simulink model "uav_control_SMC2"  (R2023a)
settings: Solver=FixedStepAuto  StartTime=0.0  StopTime=100  FixedStep=1e-3
undefined symbols (not defined in the file): c_1, c_2, c_3, c_4, c_5, c_6, c_7, c_8, c_psi, c_z, eps1, eps2, eps3, eps4, eta1, eta2, eta3, eta4, Matrix_Force2angular_velocity
libraries: simulink x18, control_form_LagrangeSimplified x1, control_form_LagrangeSimplified_forces x1
settings Model: Creator=Alex  LastModifiedBy=Alex

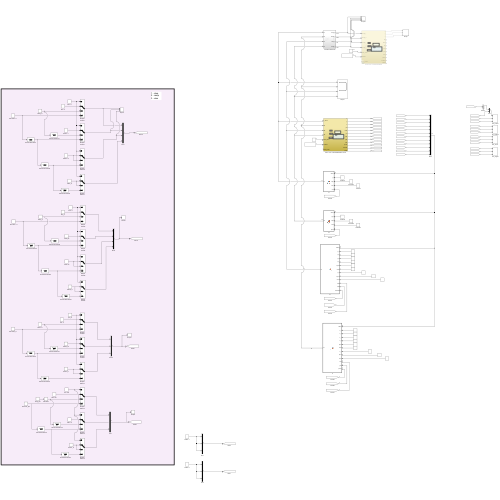
[thumbnail: Simulink's stored preview of the top-level diagram]
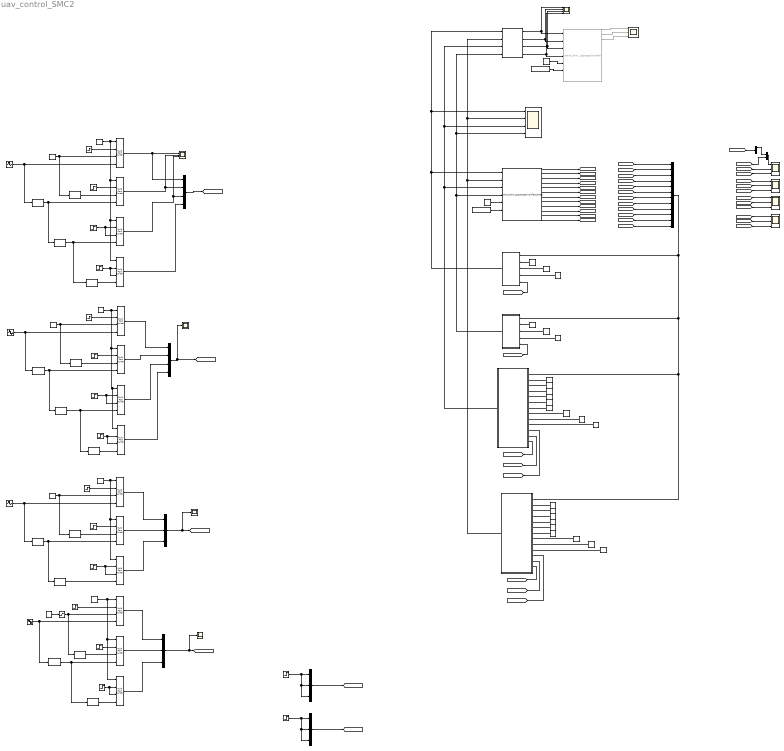
== system uav_control_SMC2 ==
  note: 1 - step
      | 2 - ramp
      | 3 - else
  CNL_AngPos : Scope  NumInputPorts=3
  CNL_AngVel : Scope  NumInputPorts=3
  CNL_LinPos : Scope  NumInputPorts=3
  CNL_LinVel : Scope  NumInputPorts=3
  Constant : Constant  Value=eta1
  Constant1 : Constant  Value=c_z
  Constant10 : Constant  Value=eps3
  Constant11 : Constant  Value=eta3
  Constant12 : Constant  Value=eps4
  Constant13 : Constant  Value=eta4
  Constant14 : Constant  Value=c_5
  Constant15 : Constant  Value=c_6
  Constant16 : Constant  Value=c_7
  Constant17 : Constant  Value=c_8
  Constant18 : Constant  Value=[1 0 0 0 1 1 0]
  Constant19 : Constant  Value=[1 1 -1 0 0 0 0 0 0 0 0 0 ]
  Constant2 : Constant  Value=eps1
  Constant20 : Constant  Value=eta1
  Constant21 : Constant  Value=c_z
  Constant22 : Constant  Value=eps1
  Constant23 : Constant  Value=eta1
  Constant24 : Constant  Value=c_z
  Constant25 : Constant  Value=eps1
  Constant26 : Constant  Value=[1 1 0 0 1 1 0]
  Constant27 : Constant  Value=[1 1 -1 0 0 0 0 0 0 0 0 0 ]
  Constant3 : Constant  Value=eta2
  Constant4 : Constant  Value=c_psi
  Constant5 : Constant  Value=eps2
  Constant6 : Constant  Value=c_1
  Constant7 : Constant  Value=c_2
  Constant8 : Constant  Value=c_3
  Constant9 : Constant  Value=c_4
  Demux : Demux
  Discrete Derivative{3..4,8..9,13..14,18..25} (14 alike) : simulink/Discrete/Discrete Derivative  gainval=1.0  ICPrevScaledInput=0.0  OutMin=[]  OutMax=[]  OutDataType=fixdt(1, 16)  OutScaling=2^-10  DoSatur=off
  Force2AngularVelocity : Subsystem
  Input_psi1 : Constant
  Input_x1 : Constant  Value=2
  Input_y1 : Constant  Value=2
  Input_z1 : Constant  Value=2
  Multiport Switch{3..4,8..9,13..14,18..25} (14 alike) : MultiPortSwitch  SaturateOnIntegerOverflow=off  InputSameDT=off
  Mux : Mux  Inputs=2
  Mux{1,3,9..10} (4 alike) : Mux  Inputs=3
  Mux2 : Mux  Inputs=12
  Mux7 : Mux
  Mux8 : Mux
  Ramp_psi1 : simulink/Sources/Ramp  slope=0.2  start=0  InitialOutput=0
  Ramp_x1 : simulink/Sources/Ramp  slope=1  start=0  InitialOutput=1
  Ramp_y1 : simulink/Sources/Ramp  slope=1  start=0  InitialOutput=0
  Ramp_z1 : simulink/Sources/Ramp  slope=-5  start=0  InitialOutput=0
  STEP0_{1..2,7..8,11..12,15..20} (12 alike) : Step  Time=0  After=0  SampleTime=0
  Saturation1 : Saturate  UpperLimit=pi  LowerLimit=-pi
  Scope : Scope  NumInputPorts=3
  Scope1 : Scope  NumInputPorts=4
  Scope2 : Scope  NumInputPorts=4
  Scope5 : Scope  NumInputPorts=3
  Scope6 : Scope
  Scope7 : Scope
  Scope8 : Scope
  Sine Wave_psi1 : Sin  SampleTime=0
  Sine Wave_x1 : Sin  Frequency=0.5  SampleTime=0
  Sine Wave_y1 : Sin  Amplitude=3  Bias=5  SampleTime=0
  Sine Wave_z1 : Sin  Amplitude=3  Bias=-5  SampleTime=0
  Step_psi1 : Step  Time=0  SampleTime=0
  Step_x1 : Step  Time=0  After=5  SampleTime=0
  Step_y1 : Step  Time=0  After=5  SampleTime=0
  Step_z1 : Step  Time=0  After=-7  SampleTime=0
  control_form_LagrangeSimplified : control_form_LagrangeSimplified/control_form_LagrangeSimplified  Commented=on  SystemSampleTime=-1  VariantActivationTime=update diagram  Latency=0  AutoFrameSizeCalculation=off
  control_form_LagrangeSimplified_forces : control_form_LagrangeSimplified_forces/control_form_LagrangeSimplified_forces  SystemSampleTime=-1  VariantActivationTime=update diagram  Latency=0  AutoFrameSizeCalculation=off
  u1 : MATLAB Function  TreatAsAtomicUnit=on
  u2 : MATLAB Function  TreatAsAtomicUnit=on
  u3 : MATLAB Function  TreatAsAtomicUnit=on
  u4 : MATLAB Function  TreatAsAtomicUnit=on
  wires:
  control_form_LagrangeSimplified_forces/1 -> [CLS_x]
  control_form_LagrangeSimplified_forces/2 -> [CLS_y]
  control_form_LagrangeSimplified_forces/3 -> [CLS_z]
  control_form_LagrangeSimplified_forces/4 -> [CLS_phi]
  control_form_LagrangeSimplified_forces/5 -> [CLS_theta]
  control_form_LagrangeSimplified_forces/6 -> [CLS_psi]
  control_form_LagrangeSimplified_forces/7 -> [CLS_xdot]
  control_form_LagrangeSimplified_forces/8 -> [CLS_ydot]
  control_form_LagrangeSimplified_forces/9 -> [CLS_zdot]
  control_form_LagrangeSimplified_forces/10 -> [CLS_phidot]
  control_form_LagrangeSimplified_forces/11 -> [CLS_thetadot]
  control_form_LagrangeSimplified_forces/12 -> [CLS_psidot]
  [CLS_x] -> Mux/2
  [CLS_y] -> CNL_LinPos/2
  [CLS_z] -> CNL_LinPos/3
  [CLS_theta] -> CNL_AngPos/2
  [CLS_phi] -> CNL_AngPos/1
  [CLS_psi] -> CNL_AngPos/3
  [CLS_xdot] -> CNL_LinVel/1
  [CLS_ydot] -> CNL_LinVel/2
  [CLS_zdot] -> CNL_LinVel/3
  [CLS_psidot] -> CNL_AngVel/3
  [CLS_thetadot] -> CNL_AngVel/2
  [CLS_phidot] -> CNL_AngVel/1
  [CLS_z] -> Mux2/3
  [CLS_psi] -> Mux2/6
  [CLS_zdot] -> Mux2/9
  [CLS_y] -> Mux2/2
  [CLS_theta] -> Mux2/5
  [CLS_ydot] -> Mux2/8
  [CLS_x] -> Mux2/1
  [CLS_phi] -> Mux2/4
  [CLS_xdot] -> Mux2/7
  [CLS_psidot] -> Mux2/12
  [CLS_thetadot] -> Mux2/11
  [CLS_phidot] -> Mux2/10
  [zref] -> u1/5(zref)
  Constant/1 -> u1/4(eta1)
  Constant1/1 -> u1/2(c_z)
  Constant2/1 -> u1/3(eps1)
  Constant5/1 -> u4/3(eps2)
  Constant4/1 -> u4/2(c_psi)
  Constant3/1 -> u4/4(eta2)
  [psiref] -> u4/5(psiref)
  Mux2/1 -> u2/1(states), u3/1(states), u4/1(states), u1/1(states)
  [xref] -> u3/12(xref)
  [thetaref] -> u3/13(thetaref)
  Constant6/1 -> u3/2(c_1)
  Constant7/1 -> u3/3(c_2)
  Constant8/1 -> u3/4(c_3)
  Constant9/1 -> u3/5(c_4)
  Constant10/1 -> u3/6(eps3)
  Constant11/1 -> u3/7(eta3)
  Constant13/1 -> u2/7(eta4)
  Constant12/1 -> u2/6(eps4)
  Constant17/1 -> u2/5(c_8)
  Constant16/1 -> u2/4(c_7)
  Constant15/1 -> u2/3(c_6)
  Constant14/1 -> u2/2(c_5)
  [phiref] -> u2/13(phiref)
  [yref] -> u2/12(yref)
  Constant18/1 -> control_form_LagrangeSimplified_forces/6
  Constant19/1 -> control_form_LagrangeSimplified_forces/5
  Multiport Switch23/1 -> Mux8/1
  Discrete Derivative9/1 -> Multiport Switch9/4, Discrete Derivative13/1
  Sine Wave_psi1/1 -> Discrete Derivative18/1, Multiport Switch14/4
  STEP0_12/1 -> Multiport Switch19/3, Multiport Switch19/2
  Multiport Switch19/1 -> Mux9/3
  Input_psi1/1 -> Multiport Switch19/1, Multiport Switch18/1, Multiport Switch14/1
  STEP0_11/1 -> Multiport Switch18/2
  Saturation1/1 -> Discrete Derivative14/1, Multiport Switch14/3
  Mux10/1 -> Scope7/1, [zref]
  Ramp_psi1/1 -> Saturation1/1
  Discrete Derivative14/1 -> Multiport Switch18/3
  Discrete Derivative23/1 -> Multiport Switch24/3
  Step_y1/1 -> Multiport Switch23/2
  Discrete Derivative18/1 -> Discrete Derivative19/1, Multiport Switch18/4
  Mux9/1 -> Scope8/1, [psiref]
  Discrete Derivative20/1 -> Discrete Derivative21/1, Multiport Switch20/4
  Step_z1/1 -> Multiport Switch8/2
  Discrete Derivative24/1 -> Discrete Derivative25/1, Multiport Switch24/4
  Multiport Switch24/1 -> Mux8/2
  Multiport Switch3/1 -> Mux7/1, Scope5/1
  Step_x1/1 -> Multiport Switch3/2
  STEP0_7/1 -> Multiport Switch4/2
  Multiport Switch4/1 -> Mux7/2, Scope5/2
  Discrete Derivative4/1 -> Multiport Switch4/4, Discrete Derivative20/1
  Discrete Derivative3/1 -> Multiport Switch4/3
  Input_x1/1 -> Multiport Switch21/1, Multiport Switch20/1, Multiport Switch4/1, Multiport Switch3/1
  Multiport Switch20/1 -> Mux7/3, Scope5/3
  Step_psi1/1 -> Multiport Switch14/2
  Mux7/1 -> [xref]
  Ramp_y1/1 -> Multiport Switch23/3, Discrete Derivative23/1
  Ramp_x1/1 -> Discrete Derivative3/1, Multiport Switch3/3
  Multiport Switch22/1 -> Mux8/4
  STEP0_15/1 -> Multiport Switch20/3, Multiport Switch20/2
  Discrete Derivative21/1 -> Multiport Switch21/4
  Discrete Derivative22/1 -> Multiport Switch22/4
  STEP0_16/1 -> Multiport Switch21/3, Multiport Switch21/2
  Multiport Switch14/1 -> Mux9/1
  Multiport Switch25/1 -> Mux8/3
  Input_y1/1 -> Multiport Switch22/1, Multiport Switch25/1, Multiport Switch24/1, Multiport Switch23/1
  Multiport Switch13/1 -> Mux10/3
  Sine Wave_y1/1 -> Discrete Derivative24/1, Multiport Switch23/4
  STEP0_19/1 -> Multiport Switch25/2, Multiport Switch25/3
  Discrete Derivative25/1 -> Discrete Derivative22/1, Multiport Switch25/4
  Discrete Derivative13/1 -> Multiport Switch13/4
  Input_z1/1 -> Multiport Switch13/1, Multiport Switch9/1, Multiport Switch8/1
  Sine Wave_x1/1 -> Multiport Switch3/4, Discrete Derivative4/1
  STEP0_20/1 -> Multiport Switch9/2
  Multiport Switch21/1 -> Mux7/4
  Ramp_z1/1 -> Discrete Derivative8/1, Multiport Switch8/3
  STEP0_18/1 -> Multiport Switch24/2
  Discrete Derivative8/1 -> Multiport Switch9/3
  Sine Wave_z1/1 -> Multiport Switch8/4, Discrete Derivative9/1
  Multiport Switch8/1 -> Mux10/1
  Discrete Derivative19/1 -> Multiport Switch19/4
  Multiport Switch18/1 -> Mux9/2
  Multiport Switch9/1 -> Mux10/2
  STEP0_8/1 -> Multiport Switch13/3, Multiport Switch13/2
  STEP0_17/1 -> Multiport Switch22/3, Multiport Switch22/2
  Mux8/1 -> [yref], Scope6/1
  STEP0_1/1 -> Mux1/2, Mux1/3, Mux1/1
  STEP0_2/1 -> Mux3/1, Mux3/2, Mux3/3
  Mux1/1 -> [thetaref]
  Mux3/1 -> [phiref]
  u1/1(u1) -> control_form_LagrangeSimplified_forces/1, Force2AngularVelocity/1(u1), Scope1/1  "u1"
  [zref] -> u3/11(zref)
  u4/1(u4) -> control_form_LagrangeSimplified_forces/4, Scope1/4, Force2AngularVelocity/4(u4)  "u4"
  Constant22/1 -> u3/9(eps1)
  Constant20/1 -> u3/10(eta1)
  Constant21/1 -> u3/8(c_z)
  Constant24/1 -> u2/8(c_z)
  Constant23/1 -> u2/10(eta1)
  Constant25/1 -> u2/9(eps1)
  [zref] -> u2/11(zref)
  u3/1(u3) -> control_form_LagrangeSimplified_forces/3, Force2AngularVelocity/3(u3), Scope1/3  "u3"
  u2/1(u2) -> control_form_LagrangeSimplified_forces/2, Scope1/2, Force2AngularVelocity/2(u2)  "u2"
  Mux/1 -> CNL_LinPos/1
  [xref] -> Demux/1
  Demux/1 -> Mux/1
  Force2AngularVelocity/1(omega_f) -> Scope2/1, control_form_LagrangeSimplified/1  "front"
  Force2AngularVelocity/2(omega_b) -> Scope2/2, control_form_LagrangeSimplified/2  "back"
  Force2AngularVelocity/3(omega_l) -> Scope2/3, control_form_LagrangeSimplified/3  "left"
  Force2AngularVelocity/4(omega_r) -> control_form_LagrangeSimplified/4, Scope2/4  "right"
  control_form_LagrangeSimplified/1 -> Scope/1
  control_form_LagrangeSimplified/2 -> Scope/2
  control_form_LagrangeSimplified/3 -> Scope/3
  Constant27/1 -> control_form_LagrangeSimplified/5
  Constant26/1 -> control_form_LagrangeSimplified/6

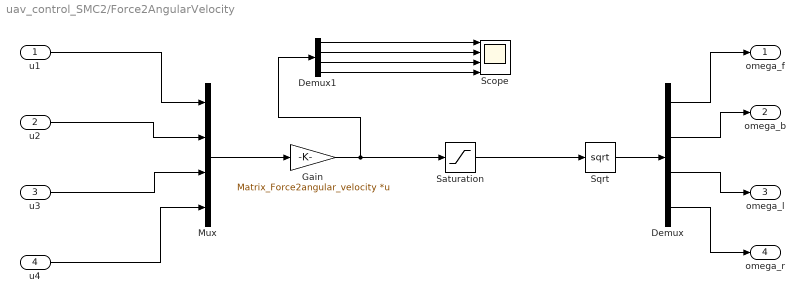
== system uav_control_SMC2/Force2AngularVelocity ==
  u1 : Inport
  u2 : Inport  Port=2
  u3 : Inport  Port=3
  u4 : Inport  Port=4
  Demux : Demux
  Demux1 : Demux
  Gain : Gain  Gain=Matrix_Force2angular_velocity  Multiplication=Matrix(K*u)
  Mux : Mux
  Saturation : Saturate  UpperLimit=inf  LowerLimit=0
  Scope : Scope  NumInputPorts=4
  Sqrt : Sqrt
  omega_f : Outport
  omega_b : Outport  Port=2
  omega_l : Outport  Port=3
  omega_r : Outport  Port=4
  wires:
  u3/1 -> Mux/3
  u2/1 -> Mux/2
  u4/1 -> Mux/4
  u1/1 -> Mux/1
  Mux/1 -> Gain/1
  Sqrt/1 -> Demux/1
  Demux/3 -> omega_l/1
  Demux/2 -> omega_b/1
  Demux/4 -> omega_r/1
  Demux/1 -> omega_f/1
  Demux1/1 -> Scope/1
  Demux1/2 -> Scope/2
  Demux1/3 -> Scope/3
  Demux1/4 -> Scope/4
  Gain/1 -> Saturation/1, Demux1/1
  Saturation/1 -> Sqrt/1

== matlab function uav_control_SMC2/u4 ==
  data: states input; c_psi input; eps2 input; eta2 input; u4 output; psiref input
function u4 = fcn_u4(states, c_psi,eps2,eta2,psiref)
    arguments
        states (12,1) {mustBeNumeric}
        c_psi
        eps2
        eta2
        psiref (3,1) {mustBeNumeric}
    end

 m=1.888;
 g=9.81;
 J1=1.453e-2;
 J2=1.453e-2;
 J3=2.884e-2;

 x=states(1);
 y=states(2);
 z=states(3);
 phi=states(4);
 theta=states(5);
 psi=states(6);
 xdot=states(7);
 ydot=states(8);
 zdot=states(9);
 phidot=states(10);
 thetadot=states(11);
 psidot=states(12);

 psidesired=psiref(1);
 psidesired_dot=psiref(2);
 psidesired_d_dot=psiref(3);
 
 s2=c_psi*(psidesired-psi)+psidesired_dot-psidot;
 u4=J3*(psidesired_d_dot-(J1-J2)/J3*phidot*thetadot+c_psi*(psidesired_dot-psidot)+eps2*sign(s2)+eta2*s2);
end

== matlab function uav_control_SMC2/u1 ==
  data: states input; c_z input; eps1 input; eta1 input; u1 output; zref input
function u1 = fcn_u1(states, c_z,eps1,eta1,zref)
    arguments
        states (12,1) {mustBeNumeric}
        c_z
        eps1
        eta1
        zref (3,1) {mustBeNumeric}
    end

 m=1.888;
 g=9.81;
 J1=1.453e-2;
 J2=1.453e-2;
 J3=2.884e-2;

 x=states(1);
 y=states(2);
 z=states(3);
 phi=states(4);
 theta=states(5);
 psi=states(6);
 xdot=states(7);
 ydot=states(8);
 zdot=states(9);
 phidot=states(10);
 thetadot=states(11);
 psidot=states(12);

 zdesired=zref(1);
 zdesired_dot=zref(2);
 zdesired_d_dot=zref(3);
 
 s1=c_z*(zdesired-z)+zdesired_dot-zdot;
 u1=m/(cos(phi)*cos(theta))*(g-zdesired_d_dot-c_z*(zdesired_dot-zdot)-eps1*saturation_f(s1/0.3)-eta1*s1);

  function out=saturation_f(x) 
    if(abs(x)<=1)
        out=x;
    else
        out=x/abs(x);
    end
end
end

== matlab function uav_control_SMC2/u3 ==
  data: states input; c_1 input; c_2 input; c_3 input; u3 output; c_4 input; eps3 input; eta3 input; c_z input; eps1 input; eta1 input; zref input; xref input; thetaref input
function u3 = fcn_u3(states, c_1,c_2,c_3,c_4,eps3,eta3,c_z, eps1, eta1, zref,xref,thetaref)
    arguments
        states (12,1) {mustBeNumeric}
        c_1
        c_2
        c_3
        c_4
        eps3
        eta3
        c_z
        eps1
        eta1
        zref
        xref (4,1) {mustBeNumeric}
        thetaref (3,1) {mustBeNumeric}
    end

 m=1.888;
 g=9.81;
 J1=1.453e-2;
 J2=1.453e-2;
 J3=2.884e-2;


 x=states(1);
 y=states(2);
 z=states(3);
 phi=states(4);
 theta=states(5);
 psi=states(6);
 xdot=states(7);
 ydot=states(8);
 zdot=states(9);
 phidot=states(10);
 thetadot=states(11);
 psidot=states(12);

 %u1
 zdesired=zref(1);
 zdesired_dot=zref(2);
 zdesired_d_dot=zref(3);
 
 s1=c_z*(zdesired-z)+zdesired_dot-zdot;
 u1=m/(cos(phi)*cos(theta))*(g-zdesired_d_dot-c_z*(zdesired_dot-zdot)-eps1*saturation_f(s1/0.3)-eta1*s1);
 
 %u3
 xdesired=xref(1);
 xdesired_dot=xref(2);
 xdesired_d_dot=xref(3);
 thetadesired=thetaref(1);
 thetadesired_dot=thetaref(2);
 thetadesired_d_dot=thetaref(3);
 x_d_dot=-1/m*(cos(phi)*sin(theta)*cos(psi)+sin(phi)*sin(psi))*u1;

 c_1=c_1/(u1*cos(phi)*cos(psi));
 c_2=c_2/(u1*cos(phi)*cos(psi));

 s3=c_1*(xdesired_dot-xdot)+c_2*(xdesired-x)+c_3*(thetadesired_dot-thetadot)+c_4*(thetadesired-theta);
 u3=J2/c_3*(thetadesired_d_dot-(J3-J1)/J2*psidot*phidot+c_4*(thetadesired_dot-thetadot)+c_2*(xdesired_dot-xdot)+c_1*(xdesired_d_dot-x_d_dot)+eps3*saturation_f(s3/0.3)+eta3*s3);
 function out=saturation_f(x) 
    if(abs(x)<=1)
        out=x;
    else
        out=x/abs(x);
    end
end
end

== matlab function uav_control_SMC2/u2 ==
  data: states input; c_5 input; c_6 input; c_7 input; u2 output; c_8 input; eps4 input; eta4 input; c_z input; eps1 input; eta1 input; zref input; yref input; phiref input
function u2 = fcn_u2(states, c_5,c_6,c_7,c_8,eps4,eta4, c_z, eps1, eta1, zref,yref,phiref)
    arguments
        states (12,1) {mustBeNumeric}
        c_5
        c_6
        c_7
        c_8
        eps4
        eta4
        c_z
        eps1
        eta1
        zref 
        yref (4,1) {mustBeNumeric}
        phiref (3,1) {mustBeNumeric}
    end

 m=1.888;
 g=9.81;
 J1=1.453e-2;
 J2=1.453e-2;
 J3=2.884e-2;

 x=states(1);
 y=states(2);
 z=states(3);
 phi=states(4);
 theta=states(5);
 psi=states(6);
 xdot=states(7);
 ydot=states(8);
 zdot=states(9);
 phidot=states(10);
 thetadot=states(11);
 psidot=states(12);
 
  %u1
 zdesired=zref(1);
 zdesired_dot=zref(2);
 zdesired_d_dot=zref(3);
 
 s1=c_z*(zdesired-z)+zdesired_dot-zdot;
 u1=m/(cos(phi)*cos(theta))*(g-zdesired_d_dot-c_z*(zdesired_dot-zdot)-eps1*saturation_f(s1/0.3)-eta1*s1);

  %u2
  ydesired=yref(1);
  ydesired_dot=yref(2);
  ydesired_d_dot=yref(3);
  phidesired=phiref(1);
  phidesired_dot=phiref(2);
  phidesired_d_dot=phiref(3);
  y_d_dot=-1/m*(cos(phi)*sin(theta)*sin(psi)-sin(phi)*cos(psi))*u1;
 
 c_5=c_5/(u1*cos(psi));
 c_6=c_6/(u1*cos(psi));

 s4=c_5*(ydesired_dot-ydot)+c_6*(ydesired-y)+c_7*(phidesired_dot-phidot)+c_8*(phidesired-phi);
 u2=J1/c_7*(phidesired_d_dot-(J2-J3)/J1*thetadot*psidot+c_8*(phidesired_dot-phidot)+c_6*(ydesired_dot-ydot)+c_5*(ydesired_d_dot-y_d_dot)+eps4*saturation_f(s4/0.3)+eta4*s4);

 function out=saturation_f(x) 
    if(abs(x)<=1)
        out=x;
    else
        out=x/abs(x);
    end
 end
end
